simulink model "lab2"  (R2018a)
settings: Solver=VariableStepAuto  StartTime=0.0  StopTime=50  RelTol=1e-3
libraries: slctrlblks x1
settings Model: Creator=vizueteharo  LastModifiedBy=Dewell
settings DebuggingCC: AlgebraicLoopMsg=none  ModelReferenceExtraNoncontSigs=none

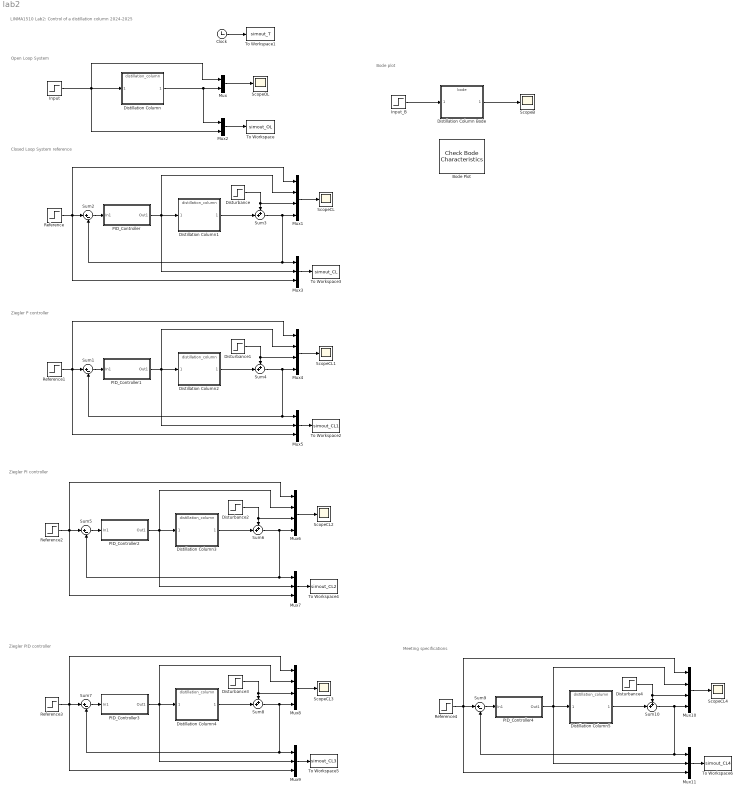
== system lab2 ==
  note: Closed Loop System reference
  note: LINMA1510 Lab2: Control of a distillation column 2024-2025
  note: Open Loop System
  note: Bode plot
  note: Ziegler P controller
  note: Ziegler PI controller
  note: Ziegler PID controller
  note: Meeting specifications
  Bode Plot : slctrlblks/Model Verification/Check Bode  Characteristics  InstantiateOnLoad=on  SaveOperatingPoints=off  LinearizationIOs={}  LinearizeAt=SnapshotTimes  SnapshotTimes=[0]  TriggerType=rising  SampleTime=auto  RateConversionMethod=zoh  PreWarpFreq=10  UseExactDelayModel=off  UseFullBlockNameLabels=off  UseBusSignalLabels=off  enabled=on  stopWhenAssertionFail=off  export=off  ViewDlgPos=[]  OpenViewOnLoad=off  LaunchViewOnOpen=off  FrequencyUnits=rad/s  MagnitudeUnits=dB  PhaseUnits=deg  TimeUnits=seconds  EnableUpperBound=off  UpperBoundFrequencies=[]  UpperBoundMagnitudes=[]  EnableLowerBound=off  LowerBoundFrequencies=[]  LowerBoundMagnitudes=[]
      settings: SourceProductName=Simulink Control Design
  Clock : Clock
  Distillation Column{,1..5} (6 alike) : ModelReference  ModelNameDialog=distillation_column  ModelReferenceVersion=1.1  CopyOfModelProtected=on
      mask Display: image('distillation_column.png');
  Distillation Column Bode : ModelReference  ModelNameDialog=bode  ModelReferenceVersion=1.2  CopyOfModelProtected=on
      mask Display: image('distillation_column.png');
  Disturbance{,1..3} (4 alike) : Step  Time=15  After=0.5  SampleTime=0
  Disturbance4 : Step  Time=0  After=0  SampleTime=0
  Input : Step  Time=0  SampleTime=0
  Input_B : Step  Time=0  SampleTime=0
  Mux : Mux  Inputs=2
  Mux{1,4,6,8,10} (5 alike) : Mux
  Mux{3,5,7,9,11} (5 alike) : Mux  Inputs=3
  Mux2 : Mux  Inputs=2
  PID_Controller : Subsystem
  PID_Controller1 : Subsystem
  PID_Controller2 : Subsystem
  PID_Controller3 : Subsystem
  PID_Controller4 : Subsystem
  Reference{,1..4} (5 alike) : Step  SampleTime=0
  ScopeB : Scope
  ScopeCL{,1..4} (5 alike) : Scope
  ScopeOL : Scope
  Sum{1..2,5,7,9} (5 alike) : Sum  Inputs=|+-
  Sum{3..4,6,8,10} (5 alike) : Sum  Inputs=++|
  To Workspace : ToWorkspace  VariableName=simout_OL  SampleTime=0.01
      settings: Save2DSignal=2-D array (concatenate along first dimension)
  To Workspace1 : ToWorkspace  VariableName=simout_T  SampleTime=0.01
      settings: Save2DSignal=2-D array (concatenate along first dimension)
  To Workspace2 : ToWorkspace  VariableName=simout_CL1  SampleTime=0.01
      settings: Save2DSignal=2-D array (concatenate along first dimension)
  To Workspace3 : ToWorkspace  VariableName=simout_CL  SampleTime=0.01
      settings: Save2DSignal=2-D array (concatenate along first dimension)
  To Workspace4 : ToWorkspace  VariableName=simout_CL2  SampleTime=0.01
      settings: Save2DSignal=2-D array (concatenate along first dimension)
  To Workspace5 : ToWorkspace  VariableName=simout_CL3  SampleTime=0.01
      settings: Save2DSignal=2-D array (concatenate along first dimension)
  To Workspace6 : ToWorkspace  VariableName=simout_CL4  SampleTime=0.01
      settings: Save2DSignal=2-D array (concatenate along first dimension)
  wires:
  Clock/1 -> To Workspace1/1
  Sum2/1 -> PID_Controller/1(In1)
  Mux1/1 -> ScopeCL/1
  Mux3/1 -> To Workspace3/1
  Distillation Column/1 -> Mux2/1, Mux/2
  Mux2/1 -> To Workspace/1
  PID_Controller/1(Out1) -> Distillation Column1/1, Mux3/2, Mux1/2
  Distillation Column1/1 -> Sum3/2
  Reference/1 -> Mux3/3, Mux1/1, Sum2/1
  Input/1 -> Mux2/2, Distillation Column/1, Mux/1
  Sum3/1 -> Sum2/2, Mux3/1, Mux1/4
  Mux/1 -> ScopeOL/1
  Disturbance/1 -> Mux1/3, Sum3/1
  Input_B/1 -> Distillation Column Bode/1
  Distillation Column Bode/1 -> ScopeB/1
  Mux5/1 -> To Workspace2/1
  Distillation Column2/1 -> Sum4/2
  Disturbance1/1 -> Mux4/3, Sum4/1
  Sum4/1 -> Sum1/2, Mux5/1, Mux4/4
  Reference1/1 -> Mux5/3, Mux4/1, Sum1/1
  PID_Controller1/1(Out1) -> Distillation Column2/1, Mux5/2, Mux4/2
  Sum1/1 -> PID_Controller1/1(In1)
  Mux4/1 -> ScopeCL1/1
  Mux6/1 -> ScopeCL2/1
  Sum5/1 -> PID_Controller2/1(In1)
  Reference2/1 -> Mux7/3, Mux6/1, Sum5/1
  PID_Controller2/1(Out1) -> Distillation Column3/1, Mux7/2, Mux6/2
  Sum6/1 -> Sum5/2, Mux7/1, Mux6/4
  Mux7/1 -> To Workspace4/1
  Disturbance2/1 -> Mux6/3, Sum6/1
  Distillation Column3/1 -> Sum6/2
  Mux8/1 -> ScopeCL3/1
  Sum7/1 -> PID_Controller3/1(In1)
  Reference3/1 -> Mux9/3, Mux8/1, Sum7/1
  PID_Controller3/1(Out1) -> Distillation Column4/1, Mux9/2, Mux8/2
  Sum8/1 -> Sum7/2, Mux9/1, Mux8/4
  Mux9/1 -> To Workspace5/1
  Disturbance3/1 -> Mux8/3, Sum8/1
  Distillation Column4/1 -> Sum8/2
  Sum10/1 -> Sum9/2, Mux11/1, Mux10/4
  Disturbance4/1 -> Mux10/3, Sum10/1
  Mux11/1 -> To Workspace6/1
  PID_Controller4/1(Out1) -> Distillation Column5/1, Mux11/2, Mux10/2
  Reference4/1 -> Mux11/3, Mux10/1, Sum9/1
  Distillation Column5/1 -> Sum10/2
  Mux10/1 -> ScopeCL4/1
  Sum9/1 -> PID_Controller4/1(In1)

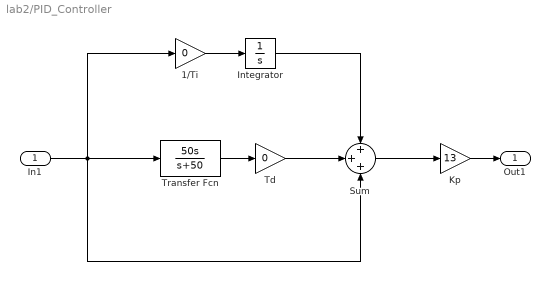
== system lab2/PID_Controller ==
  In1 : Inport
  1/Ti : Gain  Gain=0
  Integrator : Integrator
  Kp : Gain  Gain=13
  Sum : Sum  Inputs=+++
  Td : Gain  Gain=0
  Transfer Fcn : TransferFcn  Numerator=[50 0]  Denominator=[1 50]
  Out1 : Outport
  wires:
  Sum/1 -> Kp/1
  Kp/1 -> Out1/1
  1/Ti/1 -> Integrator/1
  Integrator/1 -> Sum/1
  In1/1 -> Transfer Fcn/1, Sum/3, 1/Ti/1
  Transfer Fcn/1 -> Td/1
  Td/1 -> Sum/2

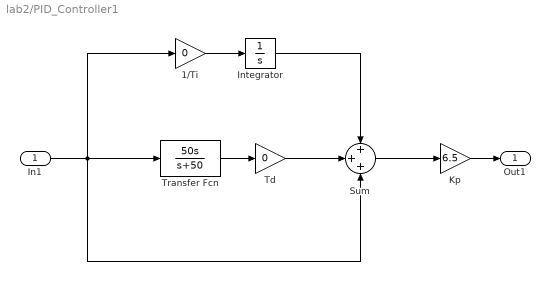
== system lab2/PID_Controller1 ==
  In1 : Inport
  1/Ti : Gain  Gain=0
  Integrator : Integrator
  Kp : Gain  Gain=6.5
  Sum : Sum  Inputs=+++
  Td : Gain  Gain=0
  Transfer Fcn : TransferFcn  Numerator=[50 0]  Denominator=[1 50]
  Out1 : Outport
  wires:
  Sum/1 -> Kp/1
  Kp/1 -> Out1/1
  1/Ti/1 -> Integrator/1
  Integrator/1 -> Sum/1
  In1/1 -> Transfer Fcn/1, Sum/3, 1/Ti/1
  Transfer Fcn/1 -> Td/1
  Td/1 -> Sum/2

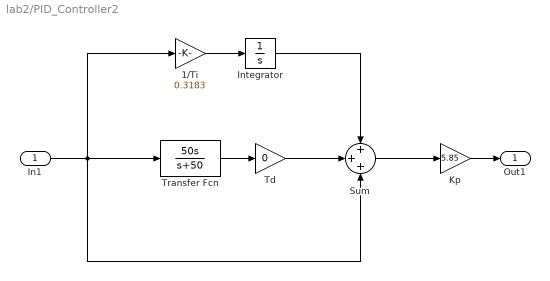
== system lab2/PID_Controller2 ==
  In1 : Inport
  1/Ti : Gain  Gain=0.3183
  Integrator : Integrator
  Kp : Gain  Gain=5.85
  Sum : Sum  Inputs=+++
  Td : Gain  Gain=0
  Transfer Fcn : TransferFcn  Numerator=[50 0]  Denominator=[1 50]
  Out1 : Outport
  wires:
  Sum/1 -> Kp/1
  Kp/1 -> Out1/1
  1/Ti/1 -> Integrator/1
  Integrator/1 -> Sum/1
  In1/1 -> Transfer Fcn/1, Sum/3, 1/Ti/1
  Transfer Fcn/1 -> Td/1
  Td/1 -> Sum/2

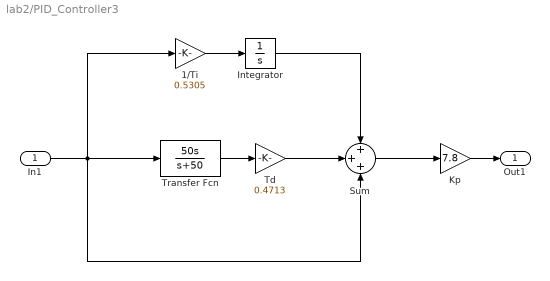
== system lab2/PID_Controller3 ==
  In1 : Inport
  1/Ti : Gain  Gain=0.5305
  Integrator : Integrator
  Kp : Gain  Gain=7.8
  Sum : Sum  Inputs=+++
  Td : Gain  Gain=0.4713
  Transfer Fcn : TransferFcn  Numerator=[50 0]  Denominator=[1 50]
  Out1 : Outport
  wires:
  Sum/1 -> Kp/1
  Kp/1 -> Out1/1
  1/Ti/1 -> Integrator/1
  Integrator/1 -> Sum/1
  In1/1 -> Transfer Fcn/1, Sum/3, 1/Ti/1
  Transfer Fcn/1 -> Td/1
  Td/1 -> Sum/2

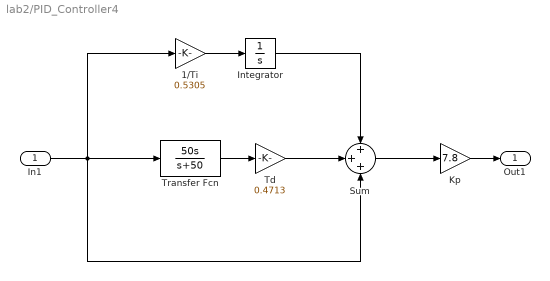
== system lab2/PID_Controller4 ==
  In1 : Inport
  1/Ti : Gain  Gain=0.5305
  Integrator : Integrator
  Kp : Gain  Gain=7.8
  Sum : Sum  Inputs=+++
  Td : Gain  Gain=0.4713
  Transfer Fcn : TransferFcn  Numerator=[50 0]  Denominator=[1 50]
  Out1 : Outport
  wires:
  Sum/1 -> Kp/1
  Kp/1 -> Out1/1
  1/Ti/1 -> Integrator/1
  Integrator/1 -> Sum/1
  In1/1 -> Transfer Fcn/1, Sum/3, 1/Ti/1
  Transfer Fcn/1 -> Td/1
  Td/1 -> Sum/2
